simulink model "Bai5b"  (R2021a)
settings: Solver=VariableStepAuto  StartTime=0.0  StopTime=10.0  RelTol=1e-3
settings Model: Creator=VTLAB  LastModifiedBy=VTLAB

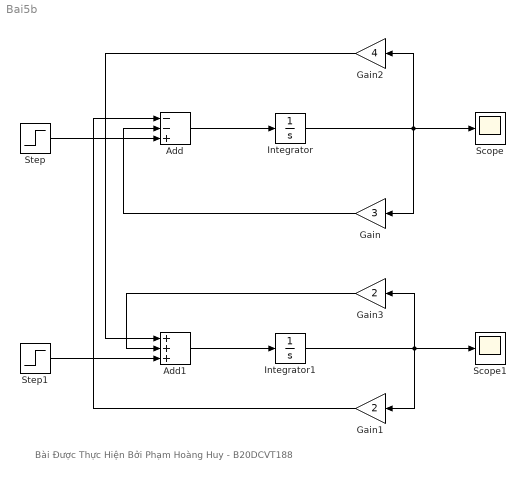
== system Bai5b ==
  note: Bài Được Thực Hiện Bởi Phạm Hoàng Huy - B20DCVT188
  Add : Sum  Inputs=--+
  Add1 : Sum  Inputs=+++
  Gain : Gain  Gain=3
  Gain1 : Gain  Gain=2
  Gain2 : Gain  Gain=4
  Gain3 : Gain  Gain=2
  Integrator : Integrator
  Integrator1 : Integrator
  Scope : Scope
  Scope1 : Scope
  Step : Step  Time=0  Before=1  SampleTime=0
  Step1 : Step  Time=0  Before=1  SampleTime=0
  wires:
  Integrator/1 -> Gain2/1, Gain/1, Scope/1
  Gain/1 -> Add/2
  Integrator1/1 -> Gain3/1, Gain1/1, Scope1/1
  Gain1/1 -> Add/1
  Gain2/1 -> Add1/1
  Gain3/1 -> Add1/2
  Add1/1 -> Integrator1/1
  Add/1 -> Integrator/1
  Step1/1 -> Add1/3
  Step/1 -> Add/3
